simulink model "verify_Entropy2_mdl"  (R2013b)
settings: Solver=VariableStepDiscrete  StartTime=0.0  StopTime=10  MaxStep=0.1  RelTol=1e-3
libraries: carnot x2, simulink x1
settings Model: Creator=drhf  LastModifiedBy=drhf
settings OptimizationCC: ExpressionDepthLimit=2147483647
settings DebuggingCC: StateNameClashWarn=warning
settings GRTTargetCC: CombineOutputUpdateFcns=off  GRTInterface=on

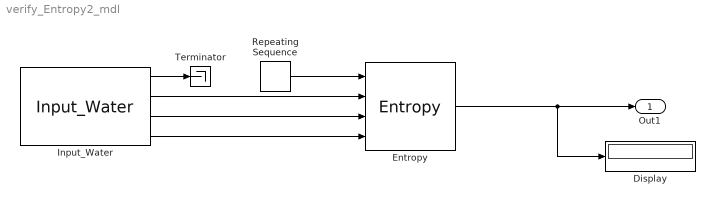
== system verify_Entropy2_mdl ==
  Display : Display
  Entropy : carnot/Basic/Material_Properties/Entropy  VariantControl=CarlibClassic  INPUTARGUMENTS=state variables (classic)  DEBUGLEVEL=WARNINGLEVEL  MAXTOTALMESSAGES=inf  MAXCONSECUTIVEMESSAGES=inf  WRITETOFILE=0  FILENAME='errors.txt'
  Input_Water : carnot/Basic/Material_Properties/Input_Water  T=20  p=2e6  xd=0
  Repeating Sequence : simulink/Sources/Repeating Sequence  rep_seq_t=[0:10 11]  rep_seq_y=[0.01 5:5:50 50]
  Terminator : Terminator
  Out1 : Outport
  wires:
  Entropy/1 -> Display/1, Out1/1
  Input_Water/4 -> Entropy/4
  Input_Water/3 -> Entropy/3
  Input_Water/1 -> Terminator/1
  Input_Water/2 -> Entropy/2
  Repeating Sequence/1 -> Entropy/1
